simulink model "UPSControl"  (R2025b)
settings: Solver=VariableStepAuto  StartTime=0.0  StopTime=10  FixedStep=Ts  RelTol=1e-3
PostLoadFcn:
  | DataCenterParam;
values from neighbouring files (symbols this model uses):
  generator = struct    [GeneratorParam.m]
  lineInductance = 1e-6    (= 1e-06)    [DataCenterParam.m]    (also in GridParam.m)
  lineResistance = 1e-3    (= 0.001)    [DataCenterParam.m]    (also in GridParam.m)
  loadPower = 5e6    (= 5000000)    [DataCenterParam.m]    (also in LVRT.m; RedundancyAnalysis.m = 10000000)
  machine = struct    [GeneratorParam.m]
  powerTau = 0.005    [DataCenterParam.m]
  Ts = 5e-5    (= 5e-05)    [DataCenterParam.m]    (also in GeneratorParam.m)
  utilizationFactor = 0.45    [DataCenterParam.m]    (also in RedundancyAnalysis.m)
undefined symbols (not defined in the file or in its folder): breaker, ctLimitDelayTime, DiscIntNeverNeededParam, ee_sli_rtmsupport, gcbh, grid, rack, ups
libraries: nesl_utility x96, fl_lib x96, eeGeneralControl x84, ee_lib x80, simulink x68, eeTransforms x30, nesl_utility_internal x16, eeSinusoidalMeasurementV2 x13, slpidlib x12, simulink_extras x12, datacenter_lib x5, batteryecm_lib x4
(part 3 of 13)

== system UPSControl/ Back up Generator/Generator Set/Detailed/Governor and Prime Mover  ==
  PRef : Inport
  Governor : Subsystem
  Ideal Torque Source : fl_lib/Mechanical/Mechanical Sources/Ideal Torque Source
  Mechanical Rotational Reference : fl_lib/Mechanical/Rotational Elements/Mechanical Rotational Reference
  Non-reheat turbine : Subsystem
  PS-Simulink Converter : nesl_utility/PS-Simulink Converter  PhysicalDomain=network_engine_domain  SubClassName=ps_output  LeftPortType=input  RightPortType=output  PseudoPeriodic=off  Frequencies=[]  VectorFormat=1-D array  Unit=1  AffineConversion=off
  Rotor Velocity Measurement : ee_lib/Electromechanical/Synchronous/Synchronous Machine Measurement  output_idx=4
      settings: InternalSimscapePortConfiguration="{\"Bottom\":[],\"Left\":[{\"id\":\"pu_input\",\"label\":\"pu\",\"type\":\"input\"}],\"Right\":[{\"id\":\"pu_output\",\"label\":\"o\",\"type\":\"output\"}],\"Top\":[]}"
  Saturation : Saturate  UpperLimit=1  LowerLimit=0
  Scope : Scope
      settings: ActiveDisplayYMinimum=-0.0012571704741974709  ActiveDisplayYMaximum=0.011314534267777241
  Scope1 : Scope
      settings: ActiveDisplayYMinimum=-1  ActiveDisplayYMaximum=1  DataLoggingVariableName=ScopeData21
  Simulink-PS Converter : nesl_utility/Simulink-PS Converter  PhysicalDomain=network_engine_domain  SubClassName=ps_input  LeftPortType=input  RightPortType=output  PseudoPeriodic=off  Frequencies=[]  NoiseDistribution=none  NoiseParameters=[]  Unit=1  AffineConversion=off  FilteringAndDerivatives=zero  SimscapeFilterOrder=1  InputFilterTimeConstant=0.001  UdotUserProvided=1
  scale by base_torque : Gain  Gain=base_torque
  R : PMIOPort  Side=Right
  C : PMIOPort  Port=2  Side=Right
  pu : PMIOPort  Port=3  Side=Left
  wires:
  PRef/1 -> Governor/2(PRef)
  scale by base_torque/1 -> Simulink-PS Converter/1
  Governor/1(delta_y) -> Non-reheat turbine/1(delta_y)
  PS-Simulink Converter/1 -> Scope1/1, Governor/1(pu_velocity)
  Non-reheat turbine/1(torque) -> Saturation/1
  Saturation/1 -> Scope/1, scale by base_torque/1
  connections:
  Simulink-PS Converter/RConn1 -- Ideal Torque Source/RConn1
  PS-Simulink Converter/LConn1 -- Rotor Velocity Measurement/RConn1
  pu/RConn1 -- Rotor Velocity Measurement/LConn1
  Ideal Torque Source/LConn1 -- R/RConn1
  Mechanical Rotational Reference/LConn1 -- Ideal Torque Source/RConn2 -- C/RConn1

== system UPSControl/ Back up Generator/Generator Set/Detailed/Measurements ==
  Current and Voltage Sensor (Three-Phase) : ee_lib/Sensors & Transducers/Current and Voltage Sensor (Three-Phase)  vMeasurementType=ee.enum.vmeasurement.lg  outputUnit=ee.enum.unit.pu  SRated=genRating*1000 A*V  VRated=Vac V  I_specify=off  I_priority=None  I=[0, 0, 0] A  I_nominal_specify=off  I_nominal_value=1  I_nominal_unit=A  V_specify=off  V_priority=None  V=[0, 0, 0] V  V_nominal_specify=off  V_nominal_value=1  V_nominal_unit=V
      settings: InternalSimscapePortConfiguration="{\"Bottom\":[],\"Left\":[{\"id\":\"N1\",\"label\":\"~1\",\"type\":\"foundation.electrical.three_phase\"}],\"Right\":[{\"id\":\"V_output\",\"label\":\"V\",\"type\":\"output\"},{\"id\":\"I_output\",\"label\":\"I\",\"type\":\"output\"},{\"id\":\"N2\",\"label\":\"~2\",\"type\":\"foundation.electrical.three_phase\"}],\"Top\":[]}"
  Gain : Gain  Gain=1/(genRating*1000)
  Gain1 : Gain  Gain=1/(genRating*1000)
  Low-Pass Filter (Discrete or Continuous)1 : eeGeneralControl/Low-Pass Filter (Discrete or Continuous)  K=1  T=0.1  B=inf  A=-inf  init_option=Inherited from block input  x0=0  Ts=-1
  Low-Pass Filter (Discrete or Continuous)2 : eeGeneralControl/Low-Pass Filter (Discrete or Continuous)  K=1  T=0.1  B=inf  A=-inf  init_option=Inherited from block input  x0=0  Ts=-1
  PLL & Measurements : Subsystem
      mask Display: image('PLL_9_7_2_20.png');
  PS-Simulink Converter{,1..3} (4 alike) : nesl_utility/PS-Simulink Converter  PhysicalDomain=network_engine_domain  SubClassName=ps_output  LeftPortType=input  RightPortType=output  PseudoPeriodic=off  Frequencies=[]  VectorFormat=inherit  Unit=inherit  AffineConversion=off
  Power Sensor (Three-Phase) : ee_lib/Sensors & Transducers/Power Sensor (Three-Phase)  load_type=ee.enum.passive.type_balanced.balanced  f0=60 Hz
      settings: InternalSimscapePortConfiguration="{\"Bottom\":[],\"Left\":[{\"id\":\"N1\",\"label\":\"~1\",\"type\":\"foundation.electrical.three_phase\"}],\"Right\":[{\"id\":\"N2\",\"label\":\"~2\",\"type\":\"foundation.electrical.three_phase\"}],\"Top\":[{\"id\":\"Pm\",\"label\":\"P\",\"type\":\"output\"},{\"id\":\"Qm\",\"label\":\"Q\",\"type\":\"output\"}]}"
  In : PMIOPort  Side=Left
  ~ : PMIOPort  Port=2  Side=Right
  P : Outport
  Q : Outport  Port=2
  V : Outport  Port=3
  I : Outport  Port=4
  wires:
  Gain1/1 -> Q/1
  Gain/1 -> P/1
  PS-Simulink Converter3/1 -> PLL & Measurements/2(I), I/1
  PS-Simulink Converter2/1 -> PLL & Measurements/1(V), V/1
  Low-Pass Filter (Discrete or Continuous)2/1 -> Gain1/1
  Low-Pass Filter (Discrete or Continuous)1/1 -> Gain/1
  PS-Simulink Converter1/1 -> Low-Pass Filter (Discrete or Continuous)2/1
  PS-Simulink Converter/1 -> Low-Pass Filter (Discrete or Continuous)1/1
  connections:
  Current and Voltage Sensor (Three-Phase)/RConn2 -- PS-Simulink Converter3/LConn1
  Current and Voltage Sensor (Three-Phase)/LConn1 -- Power Sensor (Three-Phase)/RConn1
  PS-Simulink Converter1/LConn1 -- Power Sensor (Three-Phase)/LConn3
  Current and Voltage Sensor (Three-Phase)/RConn3 -- ~/RConn1
  In/RConn1 -- Power Sensor (Three-Phase)/LConn1
  PS-Simulink Converter/LConn1 -- Power Sensor (Three-Phase)/LConn2
  Current and Voltage Sensor (Three-Phase)/RConn1 -- PS-Simulink Converter2/LConn1

== system UPSControl/ Back up Generator/Generator Set/Simplified/Exciter ==
  Current Sensor : fl_lib/Electrical/Electrical Sensors/Current Sensor
  Voltage Source : ee_lib/Sources/Voltage Source  dc_voltage=120 V  ac_voltage=0 V  ac_shift=0 rad  ac_frequency=frequency Hz  noise_mode=ee.enum.sources.noise.Disabled  PSD=0 V^2/Hz  sample_time=1e-3 s  repeatability=ee.enum.sources.repeatability.NotRepeatable  user_seed=0  auto_seed=3890346746  i_specify=off  i_priority=None  i=0 A  i_nominal_specify=off  i_nominal_value=1  i_nominal_unit=A  v_specify=off  v_priority=None  v=0 V  v_nominal_specify=off  v_nominal_value=1  v_nominal_unit=V
  + : PMIOPort  Side=Right
  - : PMIOPort  Port=2  Side=Right
  connections:
  Voltage Source/LConn1 -- Current Sensor/LConn1
  Current Sensor/RConn2 -- +/RConn1
  Voltage Source/RConn1 -- -/RConn1

== system UPSControl/ Back up Generator/Generator Set/Simplified/Measurements ==
  Current and Voltage Sensor (Three-Phase)5 : ee_lib/Sensors & Transducers/Current and Voltage Sensor (Three-Phase)  vMeasurementType=ee.enum.vmeasurement.lg  outputUnit=ee.enum.unit.pu  SRated=genRating*1000 A*V  VRated=Vac V  I_specify=off  I_priority=None  I=[0, 0, 0] A  I_nominal_specify=off  I_nominal_value=1  I_nominal_unit=A  V_specify=off  V_priority=None  V=[0, 0, 0] V  V_nominal_specify=off  V_nominal_value=1  V_nominal_unit=V
      settings: InternalSimscapePortConfiguration="{\"Bottom\":[],\"Left\":[{\"id\":\"N1\",\"label\":\"~1\",\"type\":\"foundation.electrical.three_phase\"}],\"Right\":[{\"id\":\"V_output\",\"label\":\"V\",\"type\":\"output\"},{\"id\":\"I_output\",\"label\":\"I\",\"type\":\"output\"},{\"id\":\"N2\",\"label\":\"~2\",\"type\":\"foundation.electrical.three_phase\"}],\"Top\":[]}"
  Gain : Gain  Gain=1/(genRating*1000)
  Gain1 : Gain  Gain=1/(genRating*1000)
  Low-Pass Filter (Discrete or Continuous)1 : eeGeneralControl/Low-Pass Filter (Discrete or Continuous)  K=1  T=0.1  B=inf  A=-inf  init_option=Inherited from block input  x0=0  Ts=-1
  Low-Pass Filter (Discrete or Continuous)2 : eeGeneralControl/Low-Pass Filter (Discrete or Continuous)  K=1  T=0.1  B=inf  A=-inf  init_option=Inherited from block input  x0=0  Ts=-1
  PS-Simulink Converter{,1..3} (4 alike) : nesl_utility/PS-Simulink Converter  PhysicalDomain=network_engine_domain  SubClassName=ps_output  LeftPortType=input  RightPortType=output  PseudoPeriodic=off  Frequencies=[]  VectorFormat=inherit  Unit=inherit  AffineConversion=off
  Power Sensor (Three-Phase) : ee_lib/Sensors & Transducers/Power Sensor (Three-Phase)  load_type=ee.enum.passive.type_balanced.balanced  f0=60 Hz
      settings: InternalSimscapePortConfiguration="{\"Bottom\":[],\"Left\":[{\"id\":\"N1\",\"label\":\"~1\",\"type\":\"foundation.electrical.three_phase\"}],\"Right\":[{\"id\":\"N2\",\"label\":\"~2\",\"type\":\"foundation.electrical.three_phase\"}],\"Top\":[{\"id\":\"Pm\",\"label\":\"P\",\"type\":\"output\"},{\"id\":\"Qm\",\"label\":\"Q\",\"type\":\"output\"}]}"
  In : PMIOPort  Side=Left
  ~ : PMIOPort  Port=2  Side=Right
  P : Outport
  Q : Outport  Port=2
  V : Outport  Port=3
  I : Outport  Port=4
  wires:
  Gain1/1 -> Q/1
  Gain/1 -> P/1
  PS-Simulink Converter3/1 -> I/1
  PS-Simulink Converter2/1 -> V/1
  Low-Pass Filter (Discrete or Continuous)2/1 -> Gain1/1
  Low-Pass Filter (Discrete or Continuous)1/1 -> Gain/1
  PS-Simulink Converter1/1 -> Low-Pass Filter (Discrete or Continuous)2/1
  PS-Simulink Converter/1 -> Low-Pass Filter (Discrete or Continuous)1/1
  connections:
  PS-Simulink Converter3/LConn1 -- Current and Voltage Sensor (Three-Phase)5/RConn2
  Power Sensor (Three-Phase)/RConn1 -- Current and Voltage Sensor (Three-Phase)5/LConn1
  PS-Simulink Converter1/LConn1 -- Power Sensor (Three-Phase)/LConn3
  ~/RConn1 -- Current and Voltage Sensor (Three-Phase)5/RConn3
  In/RConn1 -- Power Sensor (Three-Phase)/LConn1
  PS-Simulink Converter/LConn1 -- Power Sensor (Three-Phase)/LConn2
  PS-Simulink Converter2/LConn1 -- Current and Voltage Sensor (Three-Phase)5/RConn1

== system UPSControl/ Back up Generator/Generator Set/Simplified/Prime Mover ==
  PRef : Inport
  Ideal Torque Source : fl_lib/Mechanical/Mechanical Sources/Ideal Torque Source
  Mechanical Rotational Reference : fl_lib/Mechanical/Rotational Elements/Mechanical Rotational Reference
  Saturation : Saturate  UpperLimit=1  LowerLimit=0
  Scope : Scope
      settings: ActiveDisplayYMinimum=-1.25  ActiveDisplayYMaximum=1.25
  Simulink-PS Converter : nesl_utility/Simulink-PS Converter  PhysicalDomain=network_engine_domain  SubClassName=ps_input  LeftPortType=input  RightPortType=output  PseudoPeriodic=off  Frequencies=[]  NoiseDistribution=none  NoiseParameters=[]  Unit=1  AffineConversion=off  FilteringAndDerivatives=zero  SimscapeFilterOrder=1  InputFilterTimeConstant=0.001  UdotUserProvided=1
  scale by base_torque : Gain  Gain=genRating*1000/(2*pi*frequency)
  R : PMIOPort  Side=Right
  C : PMIOPort  Port=2  Side=Right
  wires:
  Saturation/1 -> scale by base_torque/1
  scale by base_torque/1 -> Simulink-PS Converter/1
  PRef/1 -> Scope/1, Saturation/1
  connections:
  Simulink-PS Converter/RConn1 -- Ideal Torque Source/RConn1
  Ideal Torque Source/RConn2 -- Mechanical Rotational Reference/LConn1 -- C/RConn1
  Ideal Torque Source/LConn1 -- R/RConn1

== system UPSControl/Server Load/Server Racks/PDU Racks/Server Tray ==
  AmbCPU : fl_lib/Thermal/Thermal Elements/Convective Heat Transfer  thermal_type=foundation.enum.constant_variable.constant  area=cpuSurfArea*nCPU m^2  heat_tr_coeff=htc W/(K*m^2)  min_heat_tr_coeff=1e-3 W/(K*m^2)  T_specify=off  T_priority=None  T=0 K  T_nominal_specify=off  T_nominal_value=1  T_nominal_unit=K  Q_specify=off  Q_priority=None  Q=0 W  Q_nominal_specify=off  Q_nominal_value=1  Q_nominal_unit=W
  AmbGPU : fl_lib/Thermal/Thermal Elements/Convective Heat Transfer  thermal_type=foundation.enum.constant_variable.constant  area=gpuSurfArea*nGPU m^2  heat_tr_coeff=htc W/(K*m^2)  min_heat_tr_coeff=1e-3 W/(K*m^2)  T_specify=off  T_priority=None  T=0 K  T_nominal_specify=off  T_nominal_value=1  T_nominal_unit=K  Q_specify=off  Q_priority=None  Q=0 W  Q_nominal_specify=off  Q_nominal_value=1  Q_nominal_unit=W
  PS Add : fl_lib/Physical Signals/Functions/PS Add
  Server Chip CPU : datacenter_lib/Server Chip  processorType=ProcessorType.CPU  numGPUs=4  numCPUs=nCPU  gpuTDP=1200 W  gpuIdlePower=300 W  gpuPowerExponent=1.4  hbmPowPerGPU=80 W  hbmUtilizationFrac=0.7  cpuTDP=cpuTDPperSocket W  cpuIdlePower=cpuIdlePower W  cpuPowerExponent=cpuExponent  PleakageCoeff=cpuLeakage W/K  chipTnominal=cpuNominalDieT K  chipCth=cpuDieThermalC J/K  T_specify=on  T_priority=High  T=initialT K  T_nominal_specify=off  T_nominal_value=1  T_nominal_unit=K  Q_specify=off  Q_priority=None  Q=0 W  Q_nominal_specify=off  Q_nominal_value=1  Q_nominal_unit=W
      settings: InternalSimscapePortConfiguration="{\"Bottom\":[{\"id\":\"H\",\"label\":\"H\",\"type\":\"foundation.thermal.thermal\"}],\"Left\":[{\"id\":\"U\",\"label\":\"U\",\"type\":\"input\"}],\"Right\":[{\"id\":\"Pow\",\"label\":\"P\",\"type\":\"output\"},{\"id\":\"Tchip\",\"label\":\"T\",\"type\":\"output\"}],\"Top\":[]}"
  Server Chip GPU : datacenter_lib/Server Chip  processorType=ProcessorType.GPU  numGPUs=nGPU  numCPUs=nCPU  gpuTDP=gpuTDPperDie W  gpuIdlePower=gpuIdlePower W  gpuPowerExponent=gpuExponent  hbmPowPerGPU=gpuHBMpower W  hbmUtilizationFrac=gpuHBMutil  cpuTDP=cpuTDPperSocket W  cpuIdlePower=cpuIdlePower W  cpuPowerExponent=1.1  PleakageCoeff=gpuLeakage W/K  chipTnominal=gpuNominalDieT K  chipCth=gpuDieThermalC J/K  T_specify=on  T_priority=High  T=initialT K  T_nominal_specify=off  T_nominal_value=1  T_nominal_unit=K  Q_specify=off  Q_priority=None  Q=0 W  Q_nominal_specify=off  Q_nominal_value=1  Q_nominal_unit=W
      settings: InternalSimscapePortConfiguration="{\"Bottom\":[{\"id\":\"H\",\"label\":\"H\",\"type\":\"foundation.thermal.thermal\"}],\"Left\":[{\"id\":\"U\",\"label\":\"U\",\"type\":\"input\"}],\"Right\":[{\"id\":\"Pow\",\"label\":\"P\",\"type\":\"output\"},{\"id\":\"Tchip\",\"label\":\"T\",\"type\":\"output\"}],\"Top\":[]}"
  TR_CPU_Amb : fl_lib/Thermal/Thermal Elements/Thermal Resistance  resistance=cpuAmbientR/nGPU K/W  T_specify=off  T_priority=None  T=0 K  T_nominal_specify=off  T_nominal_value=1  T_nominal_unit=K  Q_specify=off  Q_priority=None  Q=0 W  Q_nominal_specify=off  Q_nominal_value=1  Q_nominal_unit=W
  TR_CPU_substrate : fl_lib/Thermal/Thermal Elements/Thermal Resistance  resistance=cpuHeatSinkR/nGPU K/W  T_specify=off  T_priority=None  T=0 K  T_nominal_specify=off  T_nominal_value=1  T_nominal_unit=K  Q_specify=off  Q_priority=None  Q=0 W  Q_nominal_specify=off  Q_nominal_value=1  Q_nominal_unit=W
  TR_GPU_Amb : fl_lib/Thermal/Thermal Elements/Thermal Resistance  resistance=gpuAmbientR/nGPU K/W  T_specify=off  T_priority=None  T=0 K  T_nominal_specify=off  T_nominal_value=1  T_nominal_unit=K  Q_specify=off  Q_priority=None  Q=0 W  Q_nominal_specify=off  Q_nominal_value=1  Q_nominal_unit=W
  TR_GPU_substrate : fl_lib/Thermal/Thermal Elements/Thermal Resistance  resistance=gpuHeatSinkR/nGPU K/W  T_specify=off  T_priority=None  T=0 K  T_nominal_specify=off  T_nominal_value=1  T_nominal_unit=K  Q_specify=off  Q_priority=None  Q=0 W  Q_nominal_specify=off  Q_nominal_value=1  Q_nominal_unit=W
  TR_Tray_Amb : fl_lib/Thermal/Thermal Elements/Thermal Resistance  resistance=trayThermalR K/W  T_specify=off  T_priority=None  T=0 K  T_nominal_specify=off  T_nominal_value=1  T_nominal_unit=K  Q_specify=off  Q_priority=None  Q=0 W  Q_nominal_specify=off  Q_nominal_value=1  Q_nominal_unit=W
  Tray Thermal Mass : fl_lib/Thermal/Thermal Elements/Thermal Mass  mass_type=foundation.enum.constant_variable.constant  mass=trayMass kg  sp_heat=trayCp J/(K*kg)  mass_min=1e-6 kg  num_ports=foundation.enum.numPorts2.two  m_specify=off  m_priority=High  m=1 kg  m_nominal_specify=off  m_nominal_value=1  m_nominal_unit=kg  T_specify=on  T_priority=High  T=initialT K  T_nominal_specify=off  T_nominal_value=1  T_nominal_unit=K  Q_specify=off  Q_priority=None  Q=0 W  Q_nominal_specify=off  Q_nominal_value=1  Q_nominal_unit=W
      settings: InternalSimscapePortConfiguration="{\"Bottom\":[],\"Left\":[{\"id\":\"M\",\"label\":\"\",\"type\":\"foundation.thermal.thermal\"}],\"Right\":[{\"id\":\"N\",\"label\":\"\",\"type\":\"foundation.thermal.thermal\"}],\"Top\":[]}"
  U_gpu : PMIOPort  Side=Left
  U_cpu : PMIOPort  Port=2  Side=Left
  P : PMIOPort  Port=3  Side=Right
  T_gpu : PMIOPort  Port=4  Side=Right
  T_cpu : PMIOPort  Port=5  Side=Right
  Hc : PMIOPort  Port=6  Side=Right
  Ha : PMIOPort  Port=7  Side=Left
  connections:
  AmbCPU/LConn1 -- TR_CPU_Amb/RConn1
  PS Add/LConn2 -- Server Chip CPU/RConn1
  PS Add/LConn1 -- Server Chip GPU/RConn1
  P/RConn1 -- PS Add/RConn1
  Ha/RConn1 -- AmbGPU/RConn1 -- AmbCPU/RConn1
  AmbGPU/LConn1 -- TR_GPU_Amb/LConn1
  TR_Tray_Amb/RConn1 -- Hc/RConn1
  Server Chip CPU/RConn2 -- T_cpu/RConn1
  Server Chip CPU/LConn1 -- U_cpu/RConn1
  Server Chip GPU/LConn1 -- U_gpu/RConn1
  TR_Tray_Amb/LConn1 -- Tray Thermal Mass/RConn1
  TR_GPU_substrate/LConn1 -- Server Chip GPU/RConn3 -- TR_GPU_Amb/RConn1
  Server Chip CPU/RConn3 -- TR_CPU_Amb/LConn1 -- TR_CPU_substrate/LConn1
  Server Chip GPU/RConn2 -- T_gpu/RConn1
  TR_CPU_substrate/RConn1 -- TR_GPU_substrate/RConn1 -- Tray Thermal Mass/LConn1

== system UPSControl/Server Load/UPS Units/Single UPS/UPS ==
  iChrg : Inport
  DC-Link : Subsystem
      settings: CopyFcn=set_param(gcbh,'LinkStatus','none');
      mask Display: image('DCBusbattery_1.png');
  Inverter : Subsystem
      settings: PortSchema="{\"entries\":[{\"content\":{\"sides\":[{\"content\":{\"connectorIds\":[\"LConn1\",\"Out1\"]},\"type\":\"ConnectorPlacement.EquallySpacedRectSide\",\"uuid\":\"30eca24e-4a0d-4322-ab8d-7623f6b77d91\"},{\"content\":{\"connectorIds\":[\"In1\",\"RConn1\",\"RConn2\"],\"side\":\"RIGHT\"},\"type\":\"ConnectorPlacement.EquallySpacedRectSide\",\"uuid\":\"08a32252-dd7d-4c32-87e9-6b7a03d2f0b7\"},{\"content\":{\"side\":\"TOP\"},\"type\":\"ConnectorPlacement.EquallySpacedRectSide\",\"uuid\":\"b32a0ebb-b906-46f8-8fa8-e8ceac70a0fa\"}]},\"type\":\"ConnectorPlacement.EquallySpacedConnector\",\"uuid\":\"2dde14a6-acee-4d4e-9286-e85271f40ce0\"}],\"packageUris\":[\"http://schema.mathworks.com/mf0/Connector/R2020b\"],\"version\":\"1.0\"}"
      mask Display: image('Copy_2_of_Inverter.png');
  Rectifier : Subsystem
      mask Display: image('rectifier_1.png');
  ABC : PMIOPort  Side=Left
  ~ : PMIOPort  Port=2  Side=Right
  Meas : Outport
  wires:
  DC-Link/1(Meas) -> Rectifier/1(Meas), Inverter/1(DCMeas)
  Rectifier/1(Id) -> DC-Link/2(iPFC)
  iChrg/1 -> DC-Link/1(iChrg)
  Inverter/1(Meas) -> Meas/1
  Rectifier/2(V) -> DC-Link/3(vPCC)
  Rectifier/3(Brk) -> DC-Link/4(Brk)
  connections:
  Rectifier/RConn1 -- DC-Link/LConn1
  Rectifier/RConn2 -- DC-Link/LConn2
  Rectifier/LConn1 -- ABC/RConn1
  Inverter/LConn1 -- ~/RConn1
  DC-Link/RConn1 -- Inverter/RConn1
  Inverter/RConn2 -- DC-Link/RConn2

== system UPSControl/Server Load/UPS Units/Three UPS Parallel/Circuit Breaker3 ==
  BRK : Inport
  Data Type Conversion : DataTypeConversion  OutDataTypeStr=double  SaturateOnIntegerOverflow=off  RndMeth=Floor
  Open Resistance : Gain  Gain=5e6
  Phase Splitter : ee_lib/Connectors & References/Phase Splitter
  Phase Splitter1 : ee_lib/Connectors & References/Phase Splitter
  Simulink-PS Converter : nesl_utility/Simulink-PS Converter  PhysicalDomain=network_engine_domain  SubClassName=ps_input  LeftPortType=input  RightPortType=output  PseudoPeriodic=off  Frequencies=[]  NoiseDistribution=none  NoiseParameters=[]  Unit=1  AffineConversion=off  FilteringAndDerivatives=provide  SimscapeFilterOrder=1  InputFilterTimeConstant=0.001  UdotUserProvided=0
  Variable Resistor : fl_lib/Electrical/Electrical Elements/Variable Resistor  Rmin=1e-7 Ohm  thermalEnable=false  thermal_mass=1 J/K  i_specify=on  i_priority=None  i=0 A  i_nominal_specify=off  i_nominal_value=1  i_nominal_unit=A  v_specify=on  v_priority=None  v=0 V  v_nominal_specify=off  v_nominal_value=1  v_nominal_unit=V  T_specify=off  T_priority=None  T=300 K  T_nominal_specify=off  T_nominal_value=1  T_nominal_unit=K
  Variable Resistor1 : fl_lib/Electrical/Electrical Elements/Variable Resistor  Rmin=1e-7 Ohm  thermalEnable=false  thermal_mass=1 J/K  i_specify=on  i_priority=None  i=0 A  i_nominal_specify=off  i_nominal_value=1  i_nominal_unit=A  v_specify=on  v_priority=None  v=0 V  v_nominal_specify=off  v_nominal_value=1  v_nominal_unit=V  T_specify=off  T_priority=None  T=300 K  T_nominal_specify=off  T_nominal_value=1  T_nominal_unit=K
  Variable Resistor2 : fl_lib/Electrical/Electrical Elements/Variable Resistor  Rmin=1e-7 Ohm  thermalEnable=false  thermal_mass=1 J/K  i_specify=on  i_priority=None  i=0 A  i_nominal_specify=off  i_nominal_value=1  i_nominal_unit=A  v_specify=on  v_priority=None  v=0 V  v_nominal_specify=off  v_nominal_value=1  v_nominal_unit=V  T_specify=off  T_priority=None  T=300 K  T_nominal_specify=off  T_nominal_value=1  T_nominal_unit=K
  In : PMIOPort  Side=Left
  ~ : PMIOPort  Port=2  Side=Right
  wires:
  Data Type Conversion/1 -> Open Resistance/1
  BRK/1 -> Data Type Conversion/1
  Open Resistance/1 -> Simulink-PS Converter/1
  connections:
  Phase Splitter1/RConn2 -- Variable Resistor1/RConn1
  Variable Resistor1/LConn2 -- Phase Splitter/RConn2
  Phase Splitter1/RConn3 -- Variable Resistor2/RConn1
  Phase Splitter/RConn1 -- Variable Resistor/LConn2
  Variable Resistor2/LConn2 -- Phase Splitter/RConn3
  Phase Splitter1/RConn1 -- Variable Resistor/RConn1
  Phase Splitter1/LConn1 -- ~/RConn1
  Variable Resistor/LConn1 -- Simulink-PS Converter/RConn1 -- Variable Resistor2/LConn1 -- Variable Resistor1/LConn1
  Phase Splitter/LConn1 -- In/RConn1

== system UPSControl/Server Load/UPS Units/Three UPS Parallel/UPS1 ==
  iChrg : Inport
  DC-Link : Subsystem
      settings: CopyFcn=set_param(gcbh,'LinkStatus','none');
      mask Display: image('DCBusbattery_1.png');
  Inverter : Subsystem
      settings: PortSchema="{\"entries\":[{\"content\":{\"sides\":[{\"content\":{\"connectorIds\":[\"LConn1\",\"Out1\"]},\"type\":\"ConnectorPlacement.EquallySpacedRectSide\",\"uuid\":\"30eca24e-4a0d-4322-ab8d-7623f6b77d91\"},{\"content\":{\"connectorIds\":[\"In1\",\"RConn1\",\"RConn2\"],\"side\":\"RIGHT\"},\"type\":\"ConnectorPlacement.EquallySpacedRectSide\",\"uuid\":\"08a32252-dd7d-4c32-87e9-6b7a03d2f0b7\"},{\"content\":{\"side\":\"TOP\"},\"type\":\"ConnectorPlacement.EquallySpacedRectSide\",\"uuid\":\"b32a0ebb-b906-46f8-8fa8-e8ceac70a0fa\"}]},\"type\":\"ConnectorPlacement.EquallySpacedConnector\",\"uuid\":\"2dde14a6-acee-4d4e-9286-e85271f40ce0\"}],\"packageUris\":[\"http://schema.mathworks.com/mf0/Connector/R2020b\"],\"version\":\"1.0\"}"
      mask Display: image('Copy_2_of_Inverter.png');
  Rectifier : Subsystem
      mask Display: image('rectifier_1.png');
  ABC : PMIOPort  Side=Left
  ~ : PMIOPort  Port=2  Side=Right
  Meas : Outport
  wires:
  DC-Link/1(Meas) -> Rectifier/1(Meas), Inverter/1(DCMeas)
  Rectifier/1(Id) -> DC-Link/2(iPFC)
  iChrg/1 -> DC-Link/1(iChrg)
  Inverter/1(Meas) -> Meas/1
  Rectifier/2(V) -> DC-Link/3(vPCC)
  Rectifier/3(Brk) -> DC-Link/4(Brk)
  connections:
  Rectifier/RConn1 -- DC-Link/LConn1
  Rectifier/RConn2 -- DC-Link/LConn2
  Rectifier/LConn1 -- ABC/RConn1
  Inverter/LConn1 -- ~/RConn1
  DC-Link/RConn1 -- Inverter/RConn1
  Inverter/RConn2 -- DC-Link/RConn2

== system UPSControl/Server Load/UPS Units/Three UPS Parallel/UPS2 ==
  iChrg : Inport
  DC-Link : Subsystem
      settings: CopyFcn=set_param(gcbh,'LinkStatus','none');
      mask Display: image('DCBusbattery_1.png');
  Inverter : Subsystem
      settings: PortSchema="{\"entries\":[{\"content\":{\"sides\":[{\"content\":{\"connectorIds\":[\"LConn1\",\"Out1\"]},\"type\":\"ConnectorPlacement.EquallySpacedRectSide\",\"uuid\":\"30eca24e-4a0d-4322-ab8d-7623f6b77d91\"},{\"content\":{\"connectorIds\":[\"In1\",\"RConn1\",\"RConn2\"],\"side\":\"RIGHT\"},\"type\":\"ConnectorPlacement.EquallySpacedRectSide\",\"uuid\":\"08a32252-dd7d-4c32-87e9-6b7a03d2f0b7\"},{\"content\":{\"side\":\"TOP\"},\"type\":\"ConnectorPlacement.EquallySpacedRectSide\",\"uuid\":\"b32a0ebb-b906-46f8-8fa8-e8ceac70a0fa\"}]},\"type\":\"ConnectorPlacement.EquallySpacedConnector\",\"uuid\":\"2dde14a6-acee-4d4e-9286-e85271f40ce0\"}],\"packageUris\":[\"http://schema.mathworks.com/mf0/Connector/R2020b\"],\"version\":\"1.0\"}"
      mask Display: image('Copy_2_of_Inverter.png');
  Rectifier : Subsystem
      mask Display: image('rectifier_1.png');
  ABC : PMIOPort  Side=Left
  ~ : PMIOPort  Port=2  Side=Right
  Meas : Outport
  wires:
  DC-Link/1(Meas) -> Rectifier/1(Meas), Inverter/1(DCMeas)
  Rectifier/1(Id) -> DC-Link/2(iPFC)
  iChrg/1 -> DC-Link/1(iChrg)
  Inverter/1(Meas) -> Meas/1
  Rectifier/2(V) -> DC-Link/3(vPCC)
  Rectifier/3(Brk) -> DC-Link/4(Brk)
  connections:
  Rectifier/RConn1 -- DC-Link/LConn1
  Rectifier/RConn2 -- DC-Link/LConn2
  Rectifier/LConn1 -- ABC/RConn1
  Inverter/LConn1 -- ~/RConn1
  DC-Link/RConn1 -- Inverter/RConn1
  Inverter/RConn2 -- DC-Link/RConn2

== system UPSControl/Server Load/UPS Units/Three UPS Parallel/UPS3 ==
  iChrg : Inport
  DC-Link : Subsystem
      settings: CopyFcn=set_param(gcbh,'LinkStatus','none');
      mask Display: image('DCBusbattery_1.png');
  Inverter : Subsystem
      settings: PortSchema="{\"entries\":[{\"content\":{\"sides\":[{\"content\":{\"connectorIds\":[\"LConn1\",\"Out1\"]},\"type\":\"ConnectorPlacement.EquallySpacedRectSide\",\"uuid\":\"30eca24e-4a0d-4322-ab8d-7623f6b77d91\"},{\"content\":{\"connectorIds\":[\"In1\",\"RConn1\",\"RConn2\"],\"side\":\"RIGHT\"},\"type\":\"ConnectorPlacement.EquallySpacedRectSide\",\"uuid\":\"08a32252-dd7d-4c32-87e9-6b7a03d2f0b7\"},{\"content\":{\"side\":\"TOP\"},\"type\":\"ConnectorPlacement.EquallySpacedRectSide\",\"uuid\":\"b32a0ebb-b906-46f8-8fa8-e8ceac70a0fa\"}]},\"type\":\"ConnectorPlacement.EquallySpacedConnector\",\"uuid\":\"2dde14a6-acee-4d4e-9286-e85271f40ce0\"}],\"packageUris\":[\"http://schema.mathworks.com/mf0/Connector/R2020b\"],\"version\":\"1.0\"}"
      mask Display: image('Copy_2_of_Inverter.png');
  Rectifier : Subsystem
      mask Display: image('rectifier_1.png');
  ABC : PMIOPort  Side=Left
  ~ : PMIOPort  Port=2  Side=Right
  Meas : Outport
  wires:
  DC-Link/1(Meas) -> Rectifier/1(Meas), Inverter/1(DCMeas)
  Rectifier/1(Id) -> DC-Link/2(iPFC)
  iChrg/1 -> DC-Link/1(iChrg)
  Inverter/1(Meas) -> Meas/1
  Rectifier/2(V) -> DC-Link/3(vPCC)
  Rectifier/3(Brk) -> DC-Link/4(Brk)
  connections:
  Rectifier/RConn1 -- DC-Link/LConn1
  Rectifier/RConn2 -- DC-Link/LConn2
  Rectifier/LConn1 -- ABC/RConn1
  Inverter/LConn1 -- ~/RConn1
  DC-Link/RConn1 -- Inverter/RConn1
  Inverter/RConn2 -- DC-Link/RConn2

== system UPSControl/ Back up Generator/Generator Set/Detailed/Governor and Prime Mover /Governor ==
  pu_velocity : Inport
  PRef : Inport  Port=2
  1/T_G : Gain  Gain=1/T_G
  1/droop : Gain  Gain=1/(droop_percentage/100)
  Delta load setpoint : Sum  Inputs=+-|
  Delta speed : Sum  Inputs=-+
  Discrete-Time Integrator1 : DiscreteIntegrator  InitialCondition=pu_torque0  SampleTime=-1  ICPrevOutput=DiscIntNeverNeededParam  ICPrevScaledInput=DiscIntNeverNeededParam
  Scope : Scope  NumInputPorts=2
      settings: ActiveDisplayYMinimum=-1  ActiveDisplayYMaximum=1
  Scope1 : Scope  NumInputPorts=2
      settings: ActiveDisplayYMinimum=-1  ActiveDisplayYMaximum=1
  Speed_ref : Constant  Value=pu_speed_reference
  Subtract : Sum  Inputs=|+-
  delta_y : Outport  VectorParamsAs1DForOutWhenUnconnected=off
  wires:
  PRef/1 -> Delta load setpoint/1
  Discrete-Time Integrator1/1 -> Subtract/2, delta_y/1, Scope1/2
  1/T_G/1 -> Discrete-Time Integrator1/1
  Subtract/1 -> 1/T_G/1, Scope1/1
  Delta load setpoint/1 -> Subtract/1
  1/droop/1 -> Delta load setpoint/2
  pu_velocity/1 -> Delta speed/2, Scope/2
  Delta speed/1 -> 1/droop/1, Scope/1
  Speed_ref/1 -> Delta speed/1

== system UPSControl/ Back up Generator/Generator Set/Detailed/Governor and Prime Mover /Non-reheat turbine ==
  delta_y : Inport
  1/T_CH : Gain  Gain=1/T_CH
  Discrete-Time Integrator1 : DiscreteIntegrator  InitialCondition=pu_torque0  SampleTime=-1  ICPrevOutput=DiscIntNeverNeededParam  ICPrevScaledInput=DiscIntNeverNeededParam
  Scope : Scope  NumInputPorts=2
      settings: ActiveDisplayYMinimum=-1  ActiveDisplayYMaximum=1
  Sum : Sum  Inputs=|+-
  torque : Outport  VectorParamsAs1DForOutWhenUnconnected=off
  wires:
  Discrete-Time Integrator1/1 -> torque/1, Scope/1, Sum/2
  1/T_CH/1 -> Discrete-Time Integrator1/1
  Sum/1 -> 1/T_CH/1
  delta_y/1 -> Sum/1, Scope/2

== system UPSControl/ Back up Generator/Generator Set/Detailed/Measurements/PLL & Measurements ==
  V : Inport
  I : Inport  Port=2
  Measurement1 : Subsystem
  Measurement2 : Subsystem
  Subsystem : Subsystem
  Out Bus Element : Outport  PortName=VIbus  Element=Vq
  Out Bus Element1 : Outport  PortName=VIbus  Element=Vd
  Out Bus Element2 : Outport  PortName=VIbus  Element=Freq
  Out Bus Element3 : Outport  PortName=VIbus  Element=Theta
  Out Bus Element4 : Outport  PortName=VIbus  Element=Vmag
  Out Bus Element5 : Outport  PortName=VIbus  Element=Iq
  Out Bus Element6 : Outport  PortName=VIbus  Element=Id
  Out Bus Element7 : Outport  PortName=VIbus  Element=Iabc
  Out Bus Element8 : Outport  PortName=VIbus  Element=Vabc
  wires:
  Subsystem/6(Id1) -> Out Bus Element6/1
  Subsystem/7(Iq1) -> Out Bus Element5/1
  Measurement1/1(Vg) -> Subsystem/2(Iabc), Out Bus Element7/1
  I/1 -> Measurement1/1(u)
  Subsystem/1(mag) -> Out Bus Element4/1
  Measurement2/1(Vg) -> Subsystem/1(Vabc), Out Bus Element8/1
  Subsystem/4(Vd) -> Out Bus Element1/1
  Subsystem/3(angle) -> Out Bus Element3/1
  Subsystem/5(Vq) -> Out Bus Element/1
  Subsystem/2(freq) -> Out Bus Element2/1
  V/1 -> Measurement2/1(u)

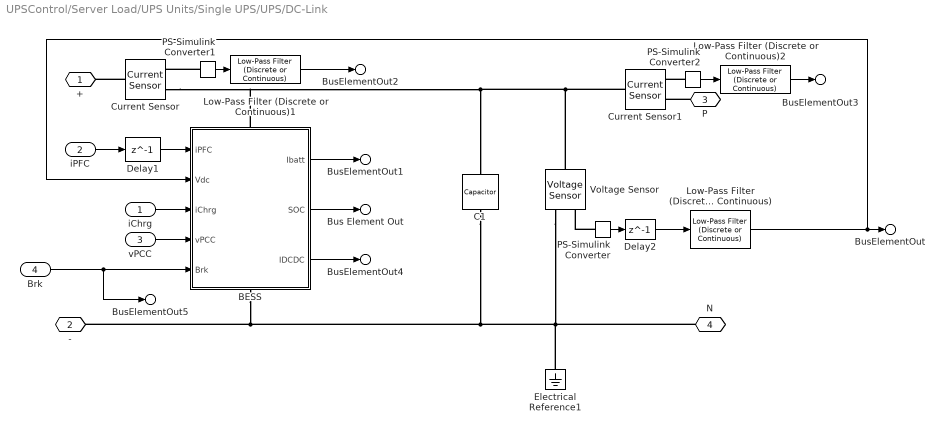
== system UPSControl/Server Load/UPS Units/Single UPS/UPS/DC-Link ==
  iChrg : Inport
  iPFC : Inport  Port=2
  vPCC : Inport  Port=3
  Brk : Inport  Port=4
  BESS : Subsystem
      settings: PortSchema="{\"entries\":[{\"content\":{\"sides\":[{\"content\":{\"connectorIds\":[\"LConn1\"]},\"type\":\"ConnectorPlacement.EquallySpacedRectSide\",\"uuid\":\"dc16109c-3681-46df-aa2d-40033a424f4f\"},{\"content\":{\"connectorIds\":[\"RConn1\"],\"side\":\"RIGHT\"},\"type\":\"ConnectorPlacement.EquallySpacedRectSide\",\"uuid\":\"5490aea4-59f2-45ea-9bac-3971cd260353\"},{\"content\":{\"connectorIds\":[\"Out1\",\"Out2\",\"Out3\"],\"side\":\"TOP\"},\"type\":\"ConnectorPlacement.EquallySpacedRectSide\",\"uuid\":\"92b5185c-680a-4a4f-a590-9680bdd408ad\"},{\"content\":{\"connectorIds\":[\"In1\",\"In2\",\"In3\",\"In4\",\"In5\"],\"side\":\"BOTTOM\"},\"type\":\"ConnectorPlacement.EquallySpacedRectSide\",\"uuid\":\"bb2f2b82-1e61-49ed-8567-aad9343e236f\"}]},\"type\":\"ConnectorPlacement.EquallySpacedConnector\",\"uuid\":\"c23d7033-d24f-41ec-a8dd-f02fcfba4177\"}],\"packageUris\":[\"http://schema.mathworks.com/mf0/Connector/R2020b\"],\"version\":\"1.0\"}"
  C1 : fl_lib/Electrical/Electrical Elements/Capacitor  c=capacitance F  r=1e-3 Ohm  g=0 1/Ohm  i_specify=on  i_priority=None  i=0 A  i_nominal_specify=off  i_nominal_value=1  i_nominal_unit=A  v_specify=off  v_priority=High  v=0 V  v_nominal_specify=off  v_nominal_value=1  v_nominal_unit=V  vc_specify=on  vc_priority=None  vc=baseVoltageDC V  vc_nominal_specify=off  vc_nominal_value=1  vc_nominal_unit=V
  Current Sensor : fl_lib/Electrical/Electrical Sensors/Current Sensor
  Current Sensor1 : fl_lib/Electrical/Electrical Sensors/Current Sensor
  Delay1 : Delay  DelayLength=1  InitialCondition=0.5
  Delay2 : Delay  DelayLength=1  InitialCondition=baseVoltageDC
  Electrical Reference1 : fl_lib/Electrical/Electrical Elements/Electrical Reference
  Low-Pass Filter (Discrete or Continuous) : eeGeneralControl/Low-Pass Filter (Discrete or Continuous)  K=1  T=0.001  B=inf  A=-inf  init_option=Inherited from block input  x0=0  Ts=-1
  Low-Pass Filter (Discrete or Continuous)1 : eeGeneralControl/Low-Pass Filter (Discrete or Continuous)  K=1  T=0.001  B=inf  A=-inf  init_option=Inherited from block input  x0=0  Ts=-1
  Low-Pass Filter (Discrete or Continuous)2 : eeGeneralControl/Low-Pass Filter (Discrete or Continuous)  K=1  T=0.001  B=inf  A=-inf  init_option=Inherited from block input  x0=0  Ts=-1
  PS-Simulink Converter : nesl_utility/PS-Simulink Converter  PhysicalDomain=network_engine_domain  SubClassName=ps_output  LeftPortType=input  RightPortType=output  PseudoPeriodic=off  Frequencies=[]  VectorFormat=inherit  Unit=inherit  AffineConversion=off
  PS-Simulink Converter1 : nesl_utility/PS-Simulink Converter  PhysicalDomain=network_engine_domain  SubClassName=ps_output  LeftPortType=input  RightPortType=output  PseudoPeriodic=off  Frequencies=[]  VectorFormat=inherit  Unit=inherit  AffineConversion=off
  PS-Simulink Converter2 : nesl_utility/PS-Simulink Converter  PhysicalDomain=network_engine_domain  SubClassName=ps_output  LeftPortType=input  RightPortType=output  PseudoPeriodic=off  Frequencies=[]  VectorFormat=inherit  Unit=inherit  AffineConversion=off
  Voltage Sensor : fl_lib/Electrical/Electrical Sensors/Voltage Sensor
  + : PMIOPort  Side=Left
  - : PMIOPort  Port=2  Side=Left
  P : PMIOPort  Port=3  Side=Right
  N : PMIOPort  Port=4  Side=Right
  Bus Element Out : Outport  PortName=Meas  Element=SOC
  BusElementOut : Outport  PortName=Meas  Element=Vdc
  BusElementOut1 : Outport  PortName=Meas  Element=Ibatt
  BusElementOut2 : Outport  PortName=Meas  Element=Idc
  BusElementOut3 : Outport  PortName=Meas  Element=ILoad
  BusElementOut4 : Outport  PortName=Meas  Element=IDCDC
  BusElementOut5 : Outport  PortName=Meas  Element=UPSBrK
  wires:
  iPFC/1 -> Delay1/1
  Delay2/1 -> Low-Pass Filter (Discrete or Continuous)/1
  iChrg/1 -> BESS/3(iChrg)
  Delay1/1 -> BESS/1(iPFC)
  PS-Simulink Converter/1 -> Delay2/1
  BESS/1(Ibatt) -> BusElementOut1/1
  vPCC/1 -> BESS/4(vPCC)
  Brk/1 -> BusElementOut5/1, BESS/5(Brk)
  BESS/2(SOC) -> Bus Element Out/1
  Low-Pass Filter (Discrete or Continuous)/1 -> BESS/2(Vdc), BusElementOut/1
  PS-Simulink Converter1/1 -> Low-Pass Filter (Discrete or Continuous)1/1
  PS-Simulink Converter2/1 -> Low-Pass Filter (Discrete or Continuous)2/1
  Low-Pass Filter (Discrete or Continuous)2/1 -> BusElementOut3/1
  Low-Pass Filter (Discrete or Continuous)1/1 -> BusElementOut2/1
  BESS/3(IDCDC) -> BusElementOut4/1
  connections:
  Electrical Reference1/LConn1 -- N/RConn1 -- Voltage Sensor/RConn2 -- C1/RConn1 -- BESS/RConn1 -- -/RConn1
  PS-Simulink Converter/LConn1 -- Voltage Sensor/RConn1
  Voltage Sensor/LConn1 -- Current Sensor1/LConn1 -- C1/LConn1 -- Current Sensor/RConn2 -- BESS/LConn1
  PS-Simulink Converter1/LConn1 -- Current Sensor/RConn1
  P/RConn1 -- Current Sensor1/RConn2
  PS-Simulink Converter2/LConn1 -- Current Sensor1/RConn1
  Current Sensor/LConn1 -- +/RConn1

== system UPSControl/Server Load/UPS Units/Single UPS/UPS/Inverter ==
  DCMeas : Inport
  DC- AC Converter : ee_lib/Semiconductors & Converters/Converters/Average-Value Voltage Source Converter (Three-Phase)  port_option=ee.enum.threePhasePort.composite  frequency_option=ee.enum.converters.frequency.variable  input_option=ee.enum.converters.inputOption.ModWave  FRated=60 Hz  losses_parameterization=ee.enum.converters.losses.fixed  Pfixed=0.5 W  ks=0.01  kc1=1.7 V  kc2=0.01 Ohm  Ploss_vect=[100, 800, 1870, 3250, 4900] W  Irms_vect=[10, 100, 200, 300, 400] A  Vdc_nom=300 V  thermal_mass=30000 J/K  temperature_specify=off  temperature_priority=High  temperature=298.15 K  temperature_nominal_specify=off  temperature_nominal_value=1  temperature_nominal_unit=K
      settings: InternalSimscapePortConfiguration="{\"Bottom\":[],\"Left\":[{\"id\":\"ModWave\",\"label\":\"ModWave\",\"type\":\"input\"},{\"id\":\"N\",\"label\":\"~\",\"type\":\"foundation.electrical.three_phase\"}],\"Right\":[{\"id\":\"p\",\"label\":\"+\",\"type\":\"foundation.electrical.electrical\"},{\"id\":\"n\",\"label\":\"-\",\"type\":\"foundation.electrical.electrical\"}],\"Top\":[]}"
  Filter & Measurements : Subsystem
      settings: PortSchema="{\"entries\":[{\"content\":{\"sides\":[{\"content\":{\"connectorIds\":[\"LConn1\",\"In1\"]},\"type\":\"ConnectorPlacement.EquallySpacedRectSide\",\"uuid\":\"460c57c7-bd36-455c-a026-acc96216539a\"},{\"content\":{\"connectorIds\":[\"Out1\",\"Out2\",\"RConn1\"],\"side\":\"RIGHT\"},\"type\":\"ConnectorPlacement.EquallySpacedRectSide\",\"uuid\":\"ae96aff3-eaea-4e67-97f2-c12a1605f490\"},{\"content\":{\"side\":\"TOP\"},\"type\":\"ConnectorPlacement.EquallySpacedRectSide\",\"uuid\":\"723b0a2f-7df5-41f2-b267-8daf9f0832d8\"}]},\"type\":\"ConnectorPlacement.EquallySpacedConnector\",\"uuid\":\"b3aac9a5-3f98-4392-99ca-65ef3ff3ee74\"}],\"packageUris\":[\"http://schema.mathworks.com/mf0/Connector/R2020b\"],\"version\":\"1.0\"}"
  Inverter Controller : Subsystem  VariantControl=Grid Forming  mask(UPS Controller){measSampleTime=ups.sampleTime, dcBusVoltage=baseVoltageDC, powerFreq=frequency, girdLineVoltage=Vac, power=plantRating*1000, fDroop=ups.inverter.fDroop, vDroop=ups.inverter.vDroop, vdPGain=ups.inverter.kpVd, VdIGain=ups.inverter.kiVd, VdMaxCt=ups.inverter.IMaxVd, VqPGain=ups.inverter.kpVq, VqIGain=ups.inverter.kiVq, VqMaxCt=ups.inverter.IMaxVd, VdMinCt=ups.inverter.IMinVd, VqMinCt=ups.inverter.IMinVd, vdvqLPFTimeConst=ups.sampleTime*100, voltControlTs=ups.sampleTime, currentControlTs=ups.sampleTime, IdPGain=ups.inverter.kpId, IdIGain=ups.inverter.kiId, IqPGain=ups.inverter.kpIq, IqIGain=ups.inverter.kiIq, filterInductance=filterInductance, currentLimitMethod=Virtual impedance, maxSatCurrentLimit=ups.iLimit.value, ctLimitXbyR=ups.iLimit.XByR, ctLimitVirtualImp=ups.iLimit.resistance}
      mask prompts: measSampleTime "Measurement sample time"; dcBusVoltage "DC bus voltage"; powerFreq "Grid frequency (Hz)"; girdLineVoltage "Grid line voltage (V)"; power "Converter power (VA)"; fDroop "Frequency droop"; vDroop "Voltage droop"; vdPGain "Vd proportional gain"; VdIGain "Vd integral gain"; VdMaxCt "Vd maximum current limit (A)"; VqPGain "Vq proportional gain"; VqIGain "Vq integral gain"; VqMaxCt "Vq maximum current limit (A)"; VdMinCt "Vd minimum current limit  (A)"; VqMinCt "Vq minimum current limit  (A)"; vdvqLPFTimeConst "Voltage measurement filter time constant (s)"; voltControlTs "Controller sample time (s)"; currentControlTs "Controller sample time (s)"; IdPGain "Id proportional gain"; IdIGain "Id integral gain"; IqPGain "Iq proportional gain"; IqIGain "Iq integral gain"; filterInductance "Filter inductance (H)"; currentLimitMethod "Current limiting method"; maxSatCurrentLimit "Maximum current limit (pu)"; ctLimitXbyR "Virtual X/R ratio"; ctLimitVirtualImp "Virtual impedance co-efficient (pu.Ohm/pu.A)"
      mask help: This block implements the uniterrupted power supply inverter control
      settings: CopyFcn=set_param(gcb,'LinkStatus','none');
      mask TypeOptions currentLimitMethod: Virtual impedance | Current saturation
      mask Callback currentLimitMethod: component.mask.iLimitSelection;
      mask DialogControl Container7 Prompt: General
      mask DialogControl Container9 Prompt: Voltage Control
      mask DialogControl Container10 Prompt: Current Control
      mask DialogControl Container8 Prompt: Current Limiting
  Simulink-PS Converter : nesl_utility/Simulink-PS Converter  PhysicalDomain=network_engine_domain  SubClassName=ps_input  LeftPortType=input  RightPortType=output  PseudoPeriodic=off  Frequencies=[]  NoiseDistribution=none  NoiseParameters=[]  Unit=1  AffineConversion=off  FilteringAndDerivatives=provide  SimscapeFilterOrder=1  InputFilterTimeConstant=0.001  UdotUserProvided=0
  ~ : PMIOPort  Side=Left
  + : PMIOPort  Port=2  Side=Right
  - : PMIOPort  Port=3  Side=Right
  Meas : Outport
  wires:
  Inverter Controller/1(mabc) -> Simulink-PS Converter/1
  DCMeas/1 -> Filter & Measurements/1(DCBusMeas)
  Filter & Measurements/1(VIBus) -> Inverter Controller/1(VI)
  Filter & Measurements/2(Meas) -> Inverter Controller/2(Power), Meas/1
  connections:
  DC- AC Converter/RConn2 -- -/RConn1
  +/RConn1 -- DC- AC Converter/RConn1
  Simulink-PS Converter/RConn1 -- DC- AC Converter/LConn1
  DC- AC Converter/LConn2 -- Filter & Measurements/LConn1
  ~/RConn1 -- Filter & Measurements/RConn1
